simulink subsystem "RegulatorCont_SubSystem"  (R2020b)
settings: Solver=VariableStepAuto  StartTime=0.0  StopTime=10.0  RelTol=1e-3
values from neighbouring files (symbols this model uses):
  A0 = A22 - L*A12    [StateSpaceControllerNominalCont.m]    (also in StateSpaceControllerNominalDigital.m; StateSpaceControllerRobustCont.m; StateSpaceControllerRobustDigital.m)
  B0 = [B2 - L*B1,(A22 - L*A12)*L+A21-L*A11]    [StateSpaceControllerNominalCont.m]    (also in StateSpaceControllerNominalDigital.m; StateSpaceControllerRobustCont.m; StateSpaceControllerRobustDigital.m)
  C0 = T*[zeros(pOutput,size(A,1) - pOutput);eye(size(A,1) - pOutput)]    [StateSpaceControllerNominalCont.m]    (also in StateSpaceControllerNominalDigital.m; StateSpaceControllerRobustCont.m; StateSpaceControllerRobustDigital.m)
  D0 = T*[zeros(pOutput,mInput),eye(pOutput);         zeros(size(A,1) - pOutput,mInput),L]    [StateSpaceControllerNominalCont.m]    (also in StateSpaceControllerNominalDigital.m; StateSpaceControllerRobustCont.m; StateSpaceControllerRobustDigital.m)
  K = place(A,B,p)    [StateSpaceControllerNominalCont.m]    (also in StateSpaceControllerNominalDigital.m; StateSpaceControllerNominalDirectDigital.m = place(Phi,Gamma,p); StateSpaceControllerRobustCont.m; StateSpaceControllerRobustDigital.m)
  Nu = reshape(Nu,[],1)    [StateSpaceControllerNominalCont.m]    (also in StateSpaceControllerNominalDigital.m; StateSpaceControllerNominalDirectDigital.m; StateSpaceControllerRobustCont.m; StateSpaceControllerRobustDigital.m)
  Nx = reshape(Nx,[],1)    [StateSpaceControllerNominalCont.m]    (also in StateSpaceControllerNominalDigital.m; StateSpaceControllerNominalDirectDigital.m; StateSpaceControllerRobustCont.m; StateSpaceControllerRobustDigital.m)
settings Model: Creator=umbe  LastModifiedBy=umbe

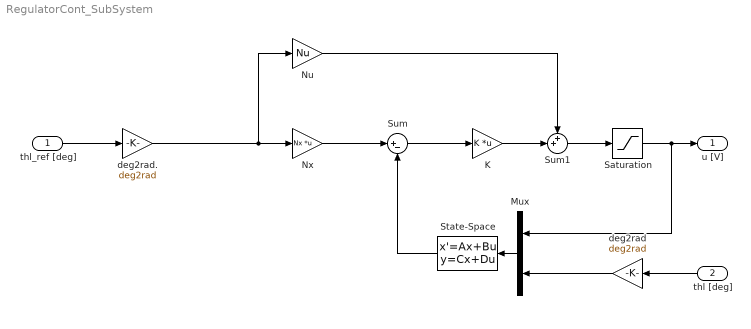
== system RegulatorCont_SubSystem ==
  thl_ref [deg] : Inport
  thl [deg] : Inport  Port=2
  K : Gain  Gain=K  Multiplication=Matrix(K*u)
  Mux : Mux  Inputs=2
  Nu : Gain  Gain=Nu
  Nx : Gain  Gain=Nx  Multiplication=Matrix(K*u)
  Saturation : Saturate  UpperLimit=10  LowerLimit=-10
  State-Space : StateSpace  A=A0  B=B0  C=C0  D=D0  InitialCondition=0
  Sum : Sum  Inputs=|+-
  Sum1 : Sum  Inputs=++|
  deg2rad : Gain  Gain=deg2rad
  deg2rad. : Gain  Gain=deg2rad
  u [V] : Outport
  wires:
  Sum1/1 -> Saturation/1
  Nu/1 -> Sum1/1
  K/1 -> Sum1/2
  Sum/1 -> K/1
  Mux/1 -> State-Space/1
  Nx/1 -> Sum/1
  deg2rad./1 -> Nx/1, Nu/1
  thl_ref [deg]/1 -> deg2rad./1
  Saturation/1 -> Mux/1, u [V]/1
  thl [deg]/1 -> deg2rad/1
  deg2rad/1 -> Mux/2
  State-Space/1 -> Sum/2
